simulink model "drone"  (R2025b)
settings: Solver=FixedStepAuto  StartTime=0.0  StopTime=3  FixedStep=0.001  MinStep=0.0005  RelTol=1e-3
libraries: Motorproplib x13, nesl_utility x4, slpidlib x4, aerolibutil x1
settings Model: SimulationMode=accelerator  Creator=cole  LastModifiedBy=cole

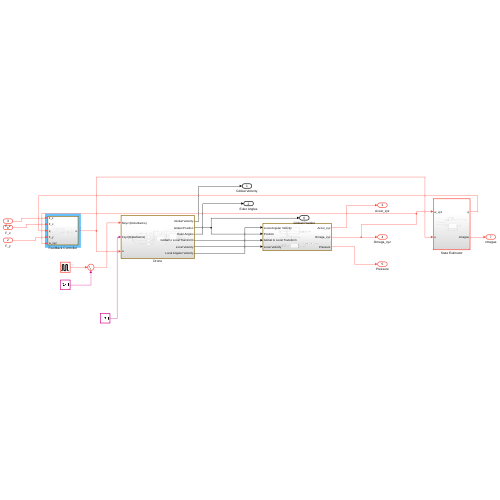
[thumbnail: Simulink's stored preview of the top-level diagram]
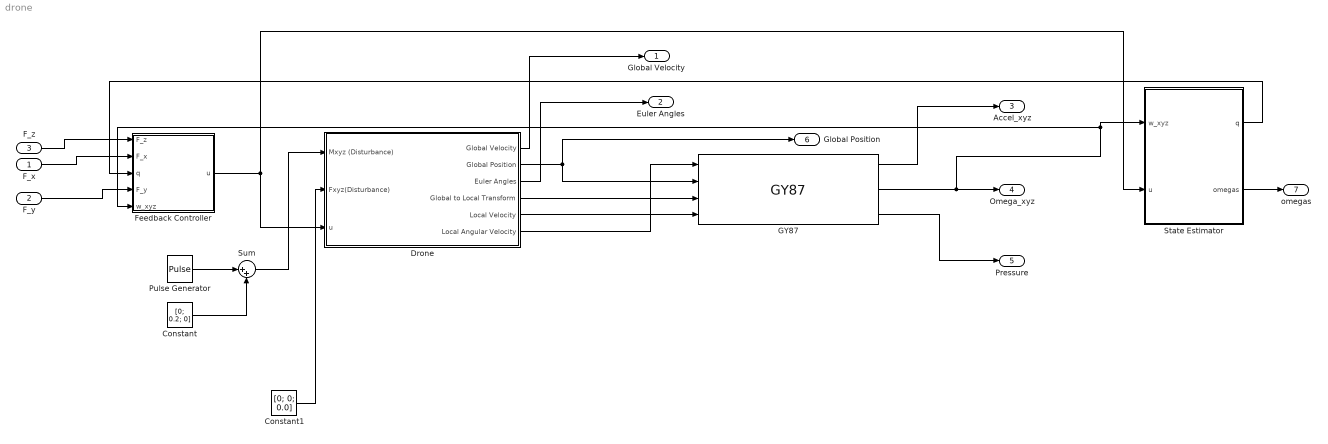
== system drone ==
  F_x : Inport
  F_y : Inport  Port=2
  F_z : Inport  Port=3
  Constant : Constant  Value=[0; 0.2; 0]
  Constant1 : Constant  Value=[0; 0; 0.0]  VectorParams1D=off
  Drone : Subsystem
  Feedback Controller : Subsystem
  GY87 : Motorproplib/GY87  SystemSampleTime=-1  VariantActivationTime=update diagram  EmptyChoice=off  PassThrough=off  PassThroughVariantControl=(default)  EmptyChoiceVariantControl=(default)  AllowFlexibleInterface=on  Latency=0  AutoFrameSizeCalculation=off
      link override Band-Limited White Noise: Cov=[0.05; 0.05; 0.05]
      link override Constant: Value=[0; 0; -9.8]
  Pulse Generator : DiscretePulseGenerator  PulseType=Time based  Amplitude=[0.0; 0.6; 0.0]  Period=10  PulseWidth=3
  State Estimator : Subsystem
  Sum : Sum  Inputs=|++
  Global Velocity : Outport
  Euler Angles : Outport  Port=2
  Accel_xyz : Outport  Port=3
  Omega_xyz : Outport  Port=4
  Pressure : Outport  Port=5
  Global Position : Outport  Port=6
  omegas : Outport  Port=7
  wires:
  Constant1/1 -> Drone/2(Fxyz(Disturbance))
  Drone/6(Local Angular Velocity) -> GY87/1
  Drone/2(Global Position) -> Global Position/1, GY87/2
  Drone/4(Global to Local Transform) -> GY87/3
  Drone/5(Local Velocity) -> GY87/4
  GY87/1 -> Accel_xyz/1
  GY87/2 -> State Estimator/1(w_xyz), Feedback Controller/5(w_xyz), Omega_xyz/1
  GY87/3 -> Pressure/1
  Drone/1(Global Velocity) -> Global Velocity/1
  State Estimator/1(q) -> Feedback Controller/3(q)
  Drone/3(Euler Angles) -> Euler Angles/1
  F_z/1 -> Feedback Controller/1(F_z)
  F_x/1 -> Feedback Controller/2(F_x)
  F_y/1 -> Feedback Controller/4(F_y)
  Feedback Controller/1(u) -> State Estimator/2(u), Drone/3(u)
  State Estimator/2(omegas) -> omegas/1
  Pulse Generator/1 -> Sum/1
  Sum/1 -> Drone/1(Mxyz (Disturbance))
  Constant/1 -> Sum/2

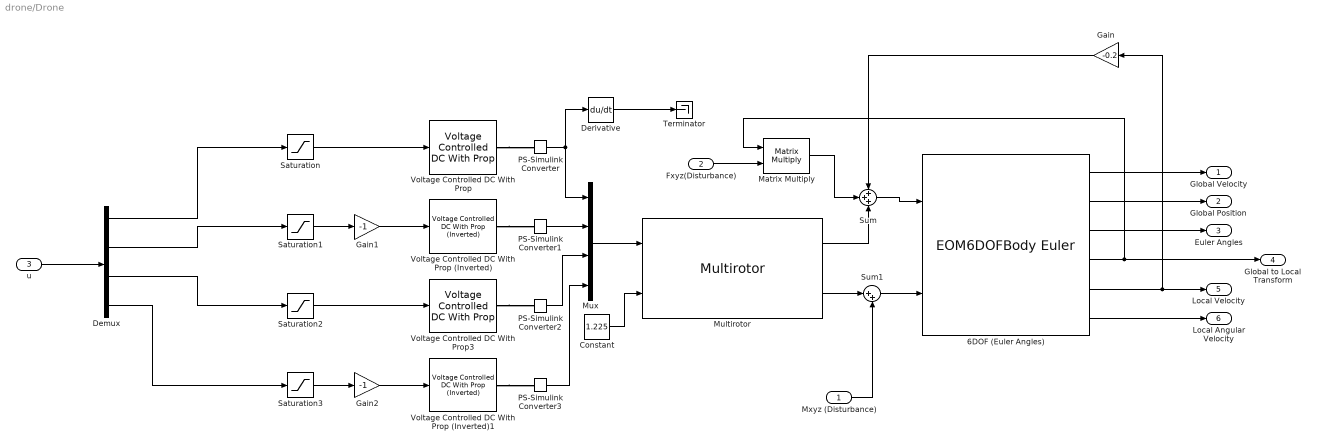
== system drone/Drone ==
  Mxyz (Disturbance) : Inport
  Fxyz(Disturbance) : Inport  Port=2
  u : Inport  Port=3
  6DOF (Euler Angles) : EOM6DOFBodyEuler  mass_0=1  inertia=[0.005194 0.0 0.0; 0.0 0.005194 0.0; 0.0 0.0 0.010296]
  Constant : Constant  Value=1.225
  Demux : Demux
  Derivative : Derivative
  Gain : Gain  Gain=-0.2
  Gain1 : Gain  Gain=-1
  Gain2 : Gain  Gain=-1
  Matrix Multiply : Product  Multiplication=Matrix(*)
  Multirotor : Multirotor  armLength=0.22  CT=0.0187  CQ=0.00446  radius=0.0635
  Mux : Mux
  PS-Simulink Converter{,1..3} (4 alike) : nesl_utility/PS-Simulink Converter  PhysicalDomain=network_engine_domain  SubClassName=ps_output  LeftPortType=input  RightPortType=output  PseudoPeriodic=off  Frequencies=[]  VectorFormat=inherit  Unit=inherit  AffineConversion=off
  Saturation{,1..3} (4 alike) : Saturate  UpperLimit=11.1  LowerLimit=0
  Sum : Sum  Inputs=+++
  Sum1 : Sum  Inputs=|++
  Terminator : Terminator
  Voltage Controlled DC With Prop : Motorproplib/Voltage Controlled DC With Prop  SystemSampleTime=-1  VariantActivationTime=update diagram  EmptyChoice=off  PassThrough=off  PassThroughVariantControl=(default)  EmptyChoiceVariantControl=(default)  AllowFlexibleInterface=on  Latency=0  AutoFrameSizeCalculation=off
  Voltage Controlled DC With Prop (Inverted) : Motorproplib/Voltage Controlled DC With Prop (Inverted)  SystemSampleTime=-1  VariantActivationTime=update diagram  EmptyChoice=off  PassThrough=off  PassThroughVariantControl=(default)  EmptyChoiceVariantControl=(default)  AllowFlexibleInterface=on  Latency=0  AutoFrameSizeCalculation=off
  Voltage Controlled DC With Prop (Inverted)1 : Motorproplib/Voltage Controlled DC With Prop (Inverted)  SystemSampleTime=-1  VariantActivationTime=update diagram  EmptyChoice=off  PassThrough=off  PassThroughVariantControl=(default)  EmptyChoiceVariantControl=(default)  AllowFlexibleInterface=on  Latency=0  AutoFrameSizeCalculation=off
  Voltage Controlled DC With Prop3 : Motorproplib/Voltage Controlled DC With Prop  SystemSampleTime=-1  VariantActivationTime=update diagram  EmptyChoice=off  PassThrough=off  PassThroughVariantControl=(default)  EmptyChoiceVariantControl=(default)  AllowFlexibleInterface=on  Latency=0  AutoFrameSizeCalculation=off
  Global Velocity : Outport
  Global Position : Outport  Port=2
  Euler Angles : Outport  Port=3
  Global to Local Transform : Outport  Port=4
  Local Velocity : Outport  Port=5
  Local Angular Velocity : Outport  Port=6
  wires:
  PS-Simulink Converter1/1 -> Mux/2
  6DOF (Euler Angles)/6 -> Local Angular Velocity/1
  6DOF (Euler Angles)/5 -> Gain/1, Local Velocity/1
  Constant/1 -> Multirotor/2
  6DOF (Euler Angles)/4 -> Matrix Multiply/1, Global to Local Transform/1
  6DOF (Euler Angles)/1 -> Global Velocity/1
  6DOF (Euler Angles)/3 -> Euler Angles/1
  PS-Simulink Converter3/1 -> Mux/4
  PS-Simulink Converter2/1 -> Mux/3
  Mux/1 -> Multirotor/1
  6DOF (Euler Angles)/2 -> Global Position/1
  PS-Simulink Converter/1 -> Derivative/1, Mux/1
  Sum/1 -> 6DOF (Euler Angles)/1
  Demux/1 -> Saturation/1
  Demux/2 -> Saturation1/1
  Multirotor/2 -> Sum1/1
  Sum1/1 -> 6DOF (Euler Angles)/2
  Mxyz (Disturbance)/1 -> Sum1/2
  Fxyz(Disturbance)/1 -> Matrix Multiply/2
  Demux/3 -> Saturation2/1
  Demux/4 -> Saturation3/1
  Multirotor/1 -> Sum/3
  Matrix Multiply/1 -> Sum/2
  Gain/1 -> Sum/1
  Derivative/1 -> Terminator/1
  Saturation/1 -> Voltage Controlled DC With Prop/1
  Saturation2/1 -> Voltage Controlled DC With Prop3/1
  Saturation3/1 -> Gain2/1
  Gain2/1 -> Voltage Controlled DC With Prop (Inverted)1/1
  Saturation1/1 -> Gain1/1
  Gain1/1 -> Voltage Controlled DC With Prop (Inverted)/1
  u/1 -> Demux/1
  connections:
  Voltage Controlled DC With Prop/RConn1 -- PS-Simulink Converter/LConn1
  Voltage Controlled DC With Prop (Inverted)/RConn1 -- PS-Simulink Converter1/LConn1
  Voltage Controlled DC With Prop3/RConn1 -- PS-Simulink Converter2/LConn1
  Voltage Controlled DC With Prop (Inverted)1/RConn1 -- PS-Simulink Converter3/LConn1

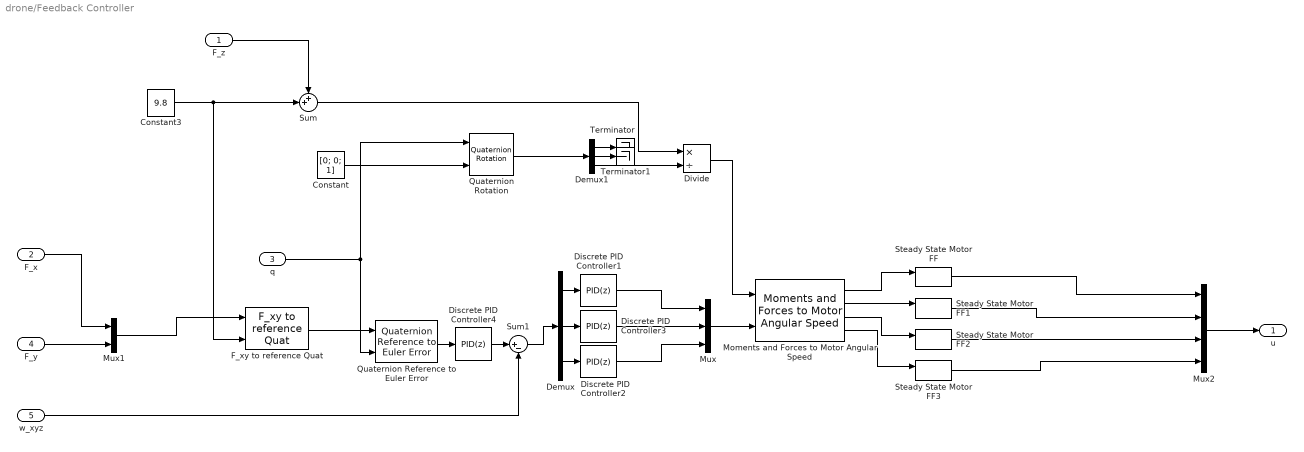
== system drone/Feedback Controller ==
  F_z : Inport
  F_x : Inport  Port=2
  q : Inport  Port=3
  F_y : Inport  Port=4
  w_xyz : Inport  Port=5
  Constant : Constant  Value=[0; 0; 1]
  Constant3 : Constant  Value=9.8
  Demux : Demux  Outputs=3
  Demux1 : Demux  Outputs=3
  Discrete PID Controller1 : slpidlib/PID Controller  Controller=PID  Form=Parallel  TimeDomain=Discrete-time  UseExternalTs=off  SampleTime=0.004  IntegratorMethod=Forward Euler  FilterMethod=Forward Euler  ControllerParametersSource=internal  P=0.2  I=0.1  UseKiTs=on  D=0.005  UseExternalDerivativeSource=off  N=80  UseFilter=off  TunerSelectOption=Transfer Function Based (PID Tuner App)  InitialConditionSource=internal  InitialConditionForIntegrator=0  InitialConditionForFilter=0  DifferentiatorICPrevScaledInput=0  ExternalReset=none  TrackingMode=off  Kt=1  LimitOutput=off  SatLimitsSource=external  UpperSaturationLimit=inf  LowerSaturationLimit=-inf  LinearizeAsGain=off  AntiWindupMode=none  Kb=1  LimitIntegrator=on  UpperIntegratorSaturationLimit=0.1  LowerIntegratorSaturationLimit=-0.1  POutMin=[]  POutMax=[]  IOutMin=[]  IOutMax=[]  DOutMin=[]  DOutMax=[]  NOutMin=[]  NOutMax=[]  SumOutMin=[]  SumOutMax=[]  SaturationOutMin=[]  SaturationOutMax=[]  PParamMin=[]  PParamMax=[]  IParamMin=[]  IParamMax=[]  DParamMin=[]  DParamMax=[]  NParamMin=[]  NParamMax=[]  KbParamMin=[]  KbParamMax=[]  KtParamMin=[]  KtParamMax=[]  KbOutMin=[]  KbOutMax=[]  KtOutMin=[]  KtOutMax=[]  IntegratorOutMin=[]  IntegratorOutMax=[]  FilterOutMin=[]  FilterOutMax=[]  SumI1OutMin=[]  SumI1OutMax=[]  SumI2OutMin=[]  SumI2OutMax=[]  SumI3OutMin=[]  SumI3OutMax=[]  SumI4OutMin=[]  SumI4OutMax=[]  SumDOutMin=[]  SumDOutMax=[]  DifferentiatorOutMin=[]  DifferentiatorOutMax=[]  FilterDiffOutCoefMin=[]  FilterDiffOutCoefMax=[]  ReciprocalOutMin=[]  ReciprocalOutMax=[]  SumDenOutMin=[]  SumDenOutMax=[]  SumNumOutMin=[]  SumNumOutMax=[]  DivideOutMin=[]  DivideOutMax=[]  UdiffTsProdOutMin=[]  UdiffTsProdOutMax=[]  NTsProdOutMin=[]  NTsProdOutMax=[]  UintegralTsProdOutMin=[]  UintegralTsProdOutMax=[]  UngainTsProdOutMin=[]  UngainTsProdOutMax=[]  ClampingZeroOutDataTypeStr=Inherit: Inherit via back propagation  ClampingZeroOutMin=[]  ClampingZeroOutMax=[]  FilterDenConstantOutDataTypeStr=Inherit: Inherit via back propagation  FilterDenConstantOutMin=[]  FilterDenConstantOutMax=[]  PCopyOutDataTypeStr=Inherit: Inherit via back propagation  PCopyOutMin=[]  PCopyOutMax=[]  NCopyOutDataTypeStr=Inherit: Inherit via back propagation  NCopyOutMin=[]  NCopyOutMax=[]  IntegratorContinuousStateAttributes=''  IntegratorStateMustResolveToSignalObject=off  IntegratorRTWStateStorageClass=Auto  FilterContinuousStateAttributes=''  FilterStateMustResolveToSignalObject=off  FilterRTWStateStorageClass=Auto  ParallelPVariant=InternalParameters  IdealPVariant=Disabled  IVariant=InternalParameters  DVariant=InternalParameters  IntegratorVariant=Discrete  SatVariant=Disabled  AWVariant=Passthrough  PCopyVariant=Disabled  TRVariant=Disabled  FdbkBlocksVariant=Forward  IdealPFdbkVariant=Disabled  SatFdbkVariant=Disabled  DerivativeFilterVariant=Differentiator  NVariant=Passthrough  NCopyVariant=Disabled_SignalSpec  FilterICVariant=InternalICsDifferentiator  IntegratorICVariant=InternalICs  ExternalResetVariant=Disabled  TRSumVariant=Passthrough  SumFdbkVariant=Disabled  SumVariant=Sum_PID  TsampFilterVariant=InternalTs  TsampNgainVariant=Passthrough  TsampIntegralVariant=Disabled_SignalSpec  ExternalSaturationOutDataTypeStr=Inherit: Same as second input  DerivativeSourceVariant=ErrorSignal  PreIntVariant=InternalPreInt
      settings: LibrarySourceBlock=simulink/Discrete/Discrete PID Controller
  Discrete PID Controller2 : slpidlib/PID Controller  Controller=PID  Form=Parallel  TimeDomain=Discrete-time  UseExternalTs=off  SampleTime=0.004  IntegratorMethod=Forward Euler  FilterMethod=Forward Euler  ControllerParametersSource=internal  P=0.04  I=0  UseKiTs=on  D=0.0  UseExternalDerivativeSource=off  N=80  UseFilter=off  TunerSelectOption=Transfer Function Based (PID Tuner App)  InitialConditionSource=internal  InitialConditionForIntegrator=0  InitialConditionForFilter=0  DifferentiatorICPrevScaledInput=0  ExternalReset=none  TrackingMode=off  Kt=1  LimitOutput=off  SatLimitsSource=internal  UpperSaturationLimit=inf  LowerSaturationLimit=-inf  LinearizeAsGain=off  AntiWindupMode=none  Kb=1  LimitIntegrator=on  UpperIntegratorSaturationLimit=0.1  LowerIntegratorSaturationLimit=-0.1  POutMin=[]  POutMax=[]  IOutMin=[]  IOutMax=[]  DOutMin=[]  DOutMax=[]  NOutMin=[]  NOutMax=[]  SumOutMin=[]  SumOutMax=[]  SaturationOutMin=[]  SaturationOutMax=[]  PParamMin=[]  PParamMax=[]  IParamMin=[]  IParamMax=[]  DParamMin=[]  DParamMax=[]  NParamMin=[]  NParamMax=[]  KbParamMin=[]  KbParamMax=[]  KtParamMin=[]  KtParamMax=[]  KbOutMin=[]  KbOutMax=[]  KtOutMin=[]  KtOutMax=[]  IntegratorOutMin=[]  IntegratorOutMax=[]  FilterOutMin=[]  FilterOutMax=[]  SumI1OutMin=[]  SumI1OutMax=[]  SumI2OutMin=[]  SumI2OutMax=[]  SumI3OutMin=[]  SumI3OutMax=[]  SumI4OutMin=[]  SumI4OutMax=[]  SumDOutMin=[]  SumDOutMax=[]  DifferentiatorOutMin=[]  DifferentiatorOutMax=[]  FilterDiffOutCoefMin=[]  FilterDiffOutCoefMax=[]  ReciprocalOutMin=[]  ReciprocalOutMax=[]  SumDenOutMin=[]  SumDenOutMax=[]  SumNumOutMin=[]  SumNumOutMax=[]  DivideOutMin=[]  DivideOutMax=[]  UdiffTsProdOutMin=[]  UdiffTsProdOutMax=[]  NTsProdOutMin=[]  NTsProdOutMax=[]  UintegralTsProdOutMin=[]  UintegralTsProdOutMax=[]  UngainTsProdOutMin=[]  UngainTsProdOutMax=[]  ClampingZeroOutDataTypeStr=Inherit: Inherit via back propagation  ClampingZeroOutMin=[]  ClampingZeroOutMax=[]  FilterDenConstantOutDataTypeStr=Inherit: Inherit via back propagation  FilterDenConstantOutMin=[]  FilterDenConstantOutMax=[]  PCopyOutDataTypeStr=Inherit: Inherit via back propagation  PCopyOutMin=[]  PCopyOutMax=[]  NCopyOutDataTypeStr=Inherit: Inherit via back propagation  NCopyOutMin=[]  NCopyOutMax=[]  IntegratorContinuousStateAttributes=''  IntegratorStateMustResolveToSignalObject=off  IntegratorRTWStateStorageClass=Auto  FilterContinuousStateAttributes=''  FilterStateMustResolveToSignalObject=off  FilterRTWStateStorageClass=Auto  ParallelPVariant=InternalParameters  IdealPVariant=Disabled  IVariant=InternalParameters  DVariant=InternalParameters  IntegratorVariant=Discrete  SatVariant=Disabled  AWVariant=Passthrough  PCopyVariant=Disabled  TRVariant=Disabled  FdbkBlocksVariant=Forward  IdealPFdbkVariant=Disabled  SatFdbkVariant=Disabled  DerivativeFilterVariant=Differentiator  NVariant=Passthrough  NCopyVariant=Disabled_SignalSpec  FilterICVariant=InternalICsDifferentiator  IntegratorICVariant=InternalICs  ExternalResetVariant=Disabled  TRSumVariant=Passthrough  SumFdbkVariant=Disabled  SumVariant=Sum_PID  TsampFilterVariant=InternalTs  TsampNgainVariant=Passthrough  TsampIntegralVariant=Disabled_SignalSpec  ExternalSaturationOutDataTypeStr=Inherit: Same as second input  DerivativeSourceVariant=ErrorSignal  PreIntVariant=InternalPreInt
      settings: LibrarySourceBlock=simulink/Discrete/Discrete PID Controller
  Discrete PID Controller3 : slpidlib/PID Controller  Controller=PID  Form=Parallel  TimeDomain=Discrete-time  UseExternalTs=off  SampleTime=0.004  IntegratorMethod=Forward Euler  FilterMethod=Forward Euler  ControllerParametersSource=internal  P=0.2  I=0.1  UseKiTs=on  D=0.005  UseExternalDerivativeSource=off  N=80  UseFilter=off  TunerSelectOption=Transfer Function Based (PID Tuner App)  InitialConditionSource=internal  InitialConditionForIntegrator=0  InitialConditionForFilter=0  DifferentiatorICPrevScaledInput=0  ExternalReset=none  TrackingMode=off  Kt=1  LimitOutput=off  SatLimitsSource=internal  UpperSaturationLimit=inf  LowerSaturationLimit=-inf  LinearizeAsGain=off  AntiWindupMode=none  Kb=1  LimitIntegrator=on  UpperIntegratorSaturationLimit=0.1  LowerIntegratorSaturationLimit=-0.1  POutMin=[]  POutMax=[]  IOutMin=[]  IOutMax=[]  DOutMin=[]  DOutMax=[]  NOutMin=[]  NOutMax=[]  SumOutMin=[]  SumOutMax=[]  SaturationOutMin=[]  SaturationOutMax=[]  PParamMin=[]  PParamMax=[]  IParamMin=[]  IParamMax=[]  DParamMin=[]  DParamMax=[]  NParamMin=[]  NParamMax=[]  KbParamMin=[]  KbParamMax=[]  KtParamMin=[]  KtParamMax=[]  KbOutMin=[]  KbOutMax=[]  KtOutMin=[]  KtOutMax=[]  IntegratorOutMin=[]  IntegratorOutMax=[]  FilterOutMin=[]  FilterOutMax=[]  SumI1OutMin=[]  SumI1OutMax=[]  SumI2OutMin=[]  SumI2OutMax=[]  SumI3OutMin=[]  SumI3OutMax=[]  SumI4OutMin=[]  SumI4OutMax=[]  SumDOutMin=[]  SumDOutMax=[]  DifferentiatorOutMin=[]  DifferentiatorOutMax=[]  FilterDiffOutCoefMin=[]  FilterDiffOutCoefMax=[]  ReciprocalOutMin=[]  ReciprocalOutMax=[]  SumDenOutMin=[]  SumDenOutMax=[]  SumNumOutMin=[]  SumNumOutMax=[]  DivideOutMin=[]  DivideOutMax=[]  UdiffTsProdOutMin=[]  UdiffTsProdOutMax=[]  NTsProdOutMin=[]  NTsProdOutMax=[]  UintegralTsProdOutMin=[]  UintegralTsProdOutMax=[]  UngainTsProdOutMin=[]  UngainTsProdOutMax=[]  ClampingZeroOutDataTypeStr=Inherit: Inherit via back propagation  ClampingZeroOutMin=[]  ClampingZeroOutMax=[]  FilterDenConstantOutDataTypeStr=Inherit: Inherit via back propagation  FilterDenConstantOutMin=[]  FilterDenConstantOutMax=[]  PCopyOutDataTypeStr=Inherit: Inherit via back propagation  PCopyOutMin=[]  PCopyOutMax=[]  NCopyOutDataTypeStr=Inherit: Inherit via back propagation  NCopyOutMin=[]  NCopyOutMax=[]  IntegratorContinuousStateAttributes=''  IntegratorStateMustResolveToSignalObject=off  IntegratorRTWStateStorageClass=Auto  FilterContinuousStateAttributes=''  FilterStateMustResolveToSignalObject=off  FilterRTWStateStorageClass=Auto  ParallelPVariant=InternalParameters  IdealPVariant=Disabled  IVariant=InternalParameters  DVariant=InternalParameters  IntegratorVariant=Discrete  SatVariant=Disabled  AWVariant=Passthrough  PCopyVariant=Disabled  TRVariant=Disabled  FdbkBlocksVariant=Forward  IdealPFdbkVariant=Disabled  SatFdbkVariant=Disabled  DerivativeFilterVariant=Differentiator  NVariant=Passthrough  NCopyVariant=Disabled_SignalSpec  FilterICVariant=InternalICsDifferentiator  IntegratorICVariant=InternalICs  ExternalResetVariant=Disabled  TRSumVariant=Passthrough  SumFdbkVariant=Disabled  SumVariant=Sum_PID  TsampFilterVariant=InternalTs  TsampNgainVariant=Passthrough  TsampIntegralVariant=Disabled_SignalSpec  ExternalSaturationOutDataTypeStr=Inherit: Same as second input  DerivativeSourceVariant=ErrorSignal  PreIntVariant=InternalPreInt
      settings: LibrarySourceBlock=simulink/Discrete/Discrete PID Controller
  Discrete PID Controller4 : slpidlib/PID Controller  Controller=PID  Form=Parallel  TimeDomain=Discrete-time  UseExternalTs=off  SampleTime=0.004  IntegratorMethod=Forward Euler  FilterMethod=Forward Euler  ControllerParametersSource=internal  P=[30.0; 30.0; 2.0]  I=[0.0; 0.0; 0.0]  UseKiTs=on  D=[0.0; 0.0; 0.0]  UseExternalDerivativeSource=off  N=80  UseFilter=off  TunerSelectOption=Transfer Function Based (PID Tuner App)  InitialConditionSource=internal  InitialConditionForIntegrator=0  InitialConditionForFilter=0  DifferentiatorICPrevScaledInput=0  ExternalReset=none  TrackingMode=off  Kt=1  LimitOutput=off  SatLimitsSource=external  UpperSaturationLimit=inf  LowerSaturationLimit=-inf  LinearizeAsGain=off  AntiWindupMode=none  Kb=1  LimitIntegrator=on  UpperIntegratorSaturationLimit=0.1  LowerIntegratorSaturationLimit=-0.1  POutMin=[]  POutMax=[]  IOutMin=[]  IOutMax=[]  DOutMin=[]  DOutMax=[]  NOutMin=[]  NOutMax=[]  SumOutMin=[]  SumOutMax=[]  SaturationOutMin=[]  SaturationOutMax=[]  PParamMin=[]  PParamMax=[]  IParamMin=[]  IParamMax=[]  DParamMin=[]  DParamMax=[]  NParamMin=[]  NParamMax=[]  KbParamMin=[]  KbParamMax=[]  KtParamMin=[]  KtParamMax=[]  KbOutMin=[]  KbOutMax=[]  KtOutMin=[]  KtOutMax=[]  IntegratorOutMin=[]  IntegratorOutMax=[]  FilterOutMin=[]  FilterOutMax=[]  SumI1OutMin=[]  SumI1OutMax=[]  SumI2OutMin=[]  SumI2OutMax=[]  SumI3OutMin=[]  SumI3OutMax=[]  SumI4OutMin=[]  SumI4OutMax=[]  SumDOutMin=[]  SumDOutMax=[]  DifferentiatorOutMin=[]  DifferentiatorOutMax=[]  FilterDiffOutCoefMin=[]  FilterDiffOutCoefMax=[]  ReciprocalOutMin=[]  ReciprocalOutMax=[]  SumDenOutMin=[]  SumDenOutMax=[]  SumNumOutMin=[]  SumNumOutMax=[]  DivideOutMin=[]  DivideOutMax=[]  UdiffTsProdOutMin=[]  UdiffTsProdOutMax=[]  NTsProdOutMin=[]  NTsProdOutMax=[]  UintegralTsProdOutMin=[]  UintegralTsProdOutMax=[]  UngainTsProdOutMin=[]  UngainTsProdOutMax=[]  ClampingZeroOutDataTypeStr=Inherit: Inherit via back propagation  ClampingZeroOutMin=[]  ClampingZeroOutMax=[]  FilterDenConstantOutDataTypeStr=Inherit: Inherit via back propagation  FilterDenConstantOutMin=[]  FilterDenConstantOutMax=[]  PCopyOutDataTypeStr=Inherit: Inherit via back propagation  PCopyOutMin=[]  PCopyOutMax=[]  NCopyOutDataTypeStr=Inherit: Inherit via back propagation  NCopyOutMin=[]  NCopyOutMax=[]  IntegratorContinuousStateAttributes=''  IntegratorStateMustResolveToSignalObject=off  IntegratorRTWStateStorageClass=Auto  FilterContinuousStateAttributes=''  FilterStateMustResolveToSignalObject=off  FilterRTWStateStorageClass=Auto  ParallelPVariant=InternalParameters  IdealPVariant=Disabled  IVariant=InternalParameters  DVariant=InternalParameters  IntegratorVariant=Discrete  SatVariant=Disabled  AWVariant=Passthrough  PCopyVariant=Disabled  TRVariant=Disabled  FdbkBlocksVariant=Forward  IdealPFdbkVariant=Disabled  SatFdbkVariant=Disabled  DerivativeFilterVariant=Differentiator  NVariant=Passthrough  NCopyVariant=Disabled_SignalSpec  FilterICVariant=InternalICsDifferentiator  IntegratorICVariant=InternalICs  ExternalResetVariant=Disabled  TRSumVariant=Passthrough  SumFdbkVariant=Disabled  SumVariant=Sum_PID  TsampFilterVariant=InternalTs  TsampNgainVariant=Passthrough  TsampIntegralVariant=Disabled_SignalSpec  ExternalSaturationOutDataTypeStr=Inherit: Same as second input  DerivativeSourceVariant=ErrorSignal  PreIntVariant=InternalPreInt
      settings: LibrarySourceBlock=simulink/Discrete/Discrete PID Controller
  Divide : Product  Inputs=*/
  F_xy to reference Quat : Motorproplib/F_xy to reference Quat  SystemSampleTime=-1  VariantActivationTime=update diagram  EmptyChoice=off  PassThrough=off  PassThroughVariantControl=(default)  EmptyChoiceVariantControl=(default)  AllowFlexibleInterface=on  Latency=0  AutoFrameSizeCalculation=off
  Moments and Forces to Motor Angular Speed : Motorproplib/Moments and Forces to Motor Angular Speed  SystemSampleTime=-1  VariantActivationTime=update diagram  EmptyChoice=off  PassThrough=off  PassThroughVariantControl=(default)  EmptyChoiceVariantControl=(default)  AllowFlexibleInterface=on  Latency=0  AutoFrameSizeCalculation=off
  Mux : Mux  Inputs=3
  Mux1 : Mux  Inputs=2
  Mux2 : Mux
  Quaternion Rotation : aerolibutil/Quaternion Rotation
  Quaternion Reference to Euler Error : Motorproplib/Quaternion Reference to Euler Error  SystemSampleTime=-1  VariantActivationTime=update diagram  EmptyChoice=off  PassThrough=off  PassThroughVariantControl=(default)  EmptyChoiceVariantControl=(default)  AllowFlexibleInterface=on  Latency=0  AutoFrameSizeCalculation=off
  Steady State Motor FF{,1..3} (4 alike) : Motorproplib/Steady State Motor FF  SystemSampleTime=-1  VariantActivationTime=update diagram  EmptyChoice=off  PassThrough=off  PassThroughVariantControl=(default)  EmptyChoiceVariantControl=(default)  AllowFlexibleInterface=on  Latency=0  AutoFrameSizeCalculation=off
  Sum : Sum  Inputs=++|
  Sum1 : Sum  Inputs=|+-
  Terminator : Terminator
  Terminator1 : Terminator
  u : Outport
  wires:
  Mux/1 -> Moments and Forces to Motor Angular Speed/2
  F_x/1 -> Mux1/1
  Moments and Forces to Motor Angular Speed/3 -> Steady State Motor FF2/1
  Demux1/2 -> Terminator1/1
  Demux/3 -> Discrete PID Controller2/1
  Demux/1 -> Discrete PID Controller1/1
  Demux/2 -> Discrete PID Controller3/1
  Constant3/1 -> Sum/2, F_xy to reference Quat/2
  Moments and Forces to Motor Angular Speed/1 -> Steady State Motor FF/1
  Steady State Motor FF3/1 -> Mux2/4
  Mux1/1 -> F_xy to reference Quat/1
  Steady State Motor FF1/1 -> Mux2/2
  q/1 -> Quaternion Reference to Euler Error/2, Quaternion Rotation/1
  Sum/1 -> Divide/1
  Constant/1 -> Quaternion Rotation/2
  F_z/1 -> Sum/1
  Moments and Forces to Motor Angular Speed/4 -> Steady State Motor FF3/1
  Divide/1 -> Moments and Forces to Motor Angular Speed/1
  Demux1/1 -> Terminator/1
  F_xy to reference Quat/1 -> Quaternion Reference to Euler Error/1
  Moments and Forces to Motor Angular Speed/2 -> Steady State Motor FF1/1
  F_y/1 -> Mux1/2
  Quaternion Rotation/1 -> Demux1/1
  Demux1/3 -> Divide/2
  w_xyz/1 -> Sum1/2
  Sum1/1 -> Demux/1
  Quaternion Reference to Euler Error/1 -> Discrete PID Controller4/1
  Discrete PID Controller4/1 -> Sum1/1
  Discrete PID Controller1/1 -> Mux/1
  Discrete PID Controller3/1 -> Mux/2
  Discrete PID Controller2/1 -> Mux/3
  Steady State Motor FF2/1 -> Mux2/3
  Steady State Motor FF/1 -> Mux2/1
  Mux2/1 -> u/1

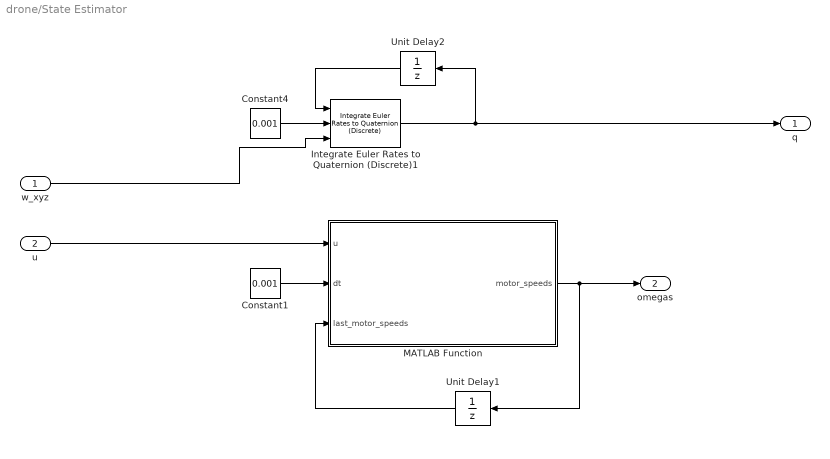
== system drone/State Estimator ==
  w_xyz : Inport
  u : Inport  Port=2
  Constant1 : Constant  Value=0.001
  Constant4 : Constant  Value=0.001
  Integrate Euler Rates to Quaternion (Discrete)1 : Motorproplib/Integrate Euler Rates to Quaternion (Discrete)  SystemSampleTime=-1  VariantActivationTime=update diagram  EmptyChoice=off  PassThrough=off  PassThroughVariantControl=(default)  EmptyChoiceVariantControl=(default)  AllowFlexibleInterface=on  Latency=0  AutoFrameSizeCalculation=off
  MATLAB Function : MATLAB Function  TreatAsAtomicUnit=on
  Unit Delay1 : UnitDelay  InitialCondition=[1; 0; 0; 0;]  SampleTime=[0.001]  HasFrameUpgradeWarning=on
  Unit Delay2 : UnitDelay  InitialCondition=[1; 0; 0; 0;]  SampleTime=[0.001]  HasFrameUpgradeWarning=on
  q : Outport
  omegas : Outport  Port=2
  wires:
  Integrate Euler Rates to Quaternion (Discrete)1/1 -> Unit Delay2/1, q/1
  MATLAB Function/1(motor_speeds) -> omegas/1, Unit Delay1/1
  Unit Delay1/1 -> MATLAB Function/3(last_motor_speeds)
  Constant1/1 -> MATLAB Function/2(dt)
  u/1 -> MATLAB Function/1(u)
  Constant4/1 -> Integrate Euler Rates to Quaternion (Discrete)1/2
  w_xyz/1 -> Integrate Euler Rates to Quaternion (Discrete)1/3
  Unit Delay2/1 -> Integrate Euler Rates to Quaternion (Discrete)1/1

== matlab function drone/State Estimator/MATLAB Function ==
  data: u input; motor_speeds output; dt input; last_motor_speeds input
function motor_speeds = fcn(u, dt, last_motor_speeds)
k_e = 0.00434058931;
R = 0.09;
k_q = 1.77354029e-8;
I_prop = 3.8e-6;

torque = (u - k_e * last_motor_speeds) / R * k_e - k_q * last_motor_speeds.^2;
motor_speeds = last_motor_speeds + torque / I_prop * dt;
